simulink model "Citation"  (Simulink 10.1)
settings: Solver=ode5  StartTime=0.0  StopTime=inf  FixedStep=0.01  RelTol=1e-3  EnableMultiTasking=on
values from neighbouring files (symbols this model uses):
  S = 12.9900    (= 12.99)    [FTFC.m]
  Vw915 = 0    [initcit.m]
  winddir = 45*(pi/180)    (= 0.785398163397)    [initcit.m]
  x0 = []    [cessnac550_3d_sfnc.m]    (also in sfunxyz.m)
undefined symbols (not defined in the file or in its folder): chord, cv1, cv2, cv3, cv4, deltagmax1, deltagmax2, deltagmax3, deltagmax4, Deng, ealphag, ealphas, g0, hDME, hGS, kt1, kt2, kt3, lh, massinit, matbuaf, matdaf, matdam, matdbbf, matdeaf, matdgaf, matdqaf, matduaf, matdwaw, matedhr, mateif, matelhr, matemhr, matemv1, matemv2, matemve, matetam, mateuaf, matfaaf, matfaxl, matff, matibaf, matibmh, matipaf, matipmh, matiraf, matiuaf, matiwaf, matlaf, matlam, matleaf, matleam, matlgaf, matlqaf, matluaf, matmaaf, matmaam, matmaf, matmam, matmbbf ... (+74)
undefined symbols (not defined in the file): matibb
libraries: simulink x12, vrlib x1
(part 5 of 5)

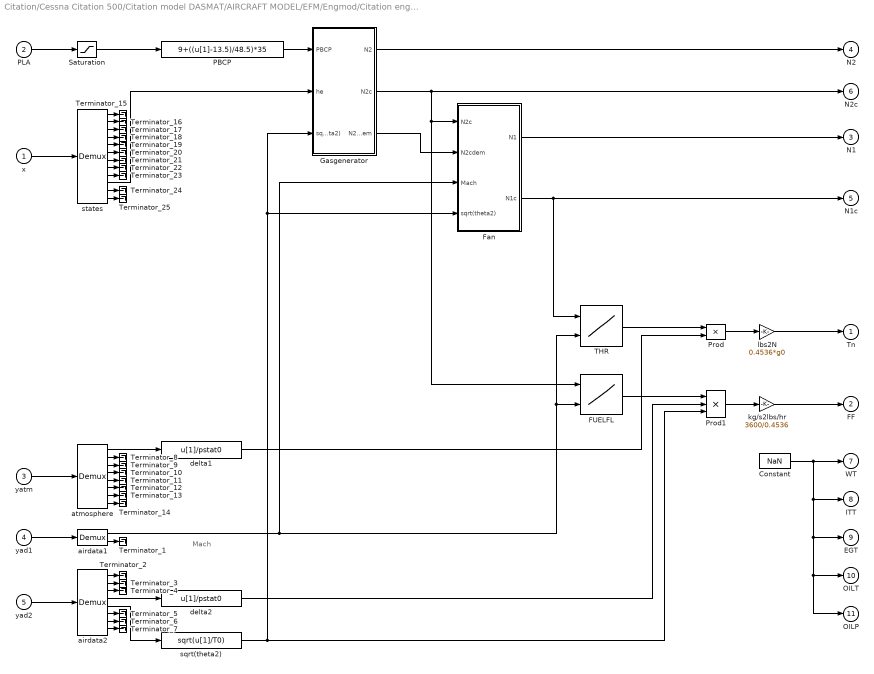
== system Citation/Cessna Citation 500/Citation model DASMAT/AIRCRAFT MODEL/EFM/Engmod/Citation eng_mod/Subsystem1/JT15 Dynamic/Subsystem/engine ==
  note: Mach
  x : Inport
  PLA : Inport  Port=2
  yatm : Inport  Port=3
  yad1 : Inport  Port=4
  yad2 : Inport  Port=5
  Constant : Constant  Value=NaN
  FUELFL : Lookup2D  RowIndex=matff(2:14,1)  ColumnIndex=matff(1,2:14)  Table=matff(2:14,2:14)  SaturateOnIntegerOverflow=on  InputSameDT=on
  Fan : Subsystem
  Gasgenerator : Subsystem
  PBCP : Fcn  Expr=9+((u[1]-13.5)/48.5)*35
  Prod : Product  InputSameDT=on  SaturateOnIntegerOverflow=on  OutDataTypeStr=Inherit: Same as first input
  Prod1 : Product  Inputs=3  InputSameDT=on  SaturateOnIntegerOverflow=on  OutDataTypeStr=Inherit: Same as first input
  Saturation : Saturate  UpperLimit=62  LowerLimit=13.5
  THR : Lookup2D  RowIndex=matthr(2:12,1)  ColumnIndex=matthr(1,2:12)  Table=matthr(2:12,2:12)  SaturateOnIntegerOverflow=on  InputSameDT=on
  Terminator_{1..25} (25 alike) : Terminator
  airdata1 : Demux  Outputs=2
      settings: DisplayOption=none
  airdata2 : Demux  Outputs=8
      settings: DisplayOption=none
  atmosphere : Demux  Outputs=8
      settings: DisplayOption=none
  delta1 : Fcn  Expr=u[1]/pstat0
  delta2 : Fcn  Expr=u[1]/pstat0
  kg/s2lbs/hr : Gain  Gain=3600/0.4536  SaturateOnIntegerOverflow=on  OutDataTypeStr=Inherit: Same as input  ParamDataTypeStr=Inherit: Same as input
  lbs2N : Gain  Gain=0.4536*g0  SaturateOnIntegerOverflow=on  OutDataTypeStr=Inherit: Same as input  ParamDataTypeStr=Inherit: Same as input
  sqrt(theta2) : Fcn  Expr=sqrt(u[1]/T0)
  states : Demux  Outputs=12
      settings: DisplayOption=none
  Tn : Outport
  FF : Outport  Port=2
  N1 : Outport  Port=3
  N2 : Outport  Port=4
  N1c : Outport  Port=5
  N2c : Outport  Port=6
  WT : Outport  Port=7
  ITT : Outport  Port=8
  EGT : Outport  Port=9
  OILT : Outport  Port=10
  OILP : Outport  Port=11
  wires:
  states/12 -> Terminator_25/1
  states/11 -> Terminator_24/1
  states/9 -> Terminator_23/1
  states/8 -> Terminator_22/1
  states/7 -> Terminator_21/1
  states/6 -> Terminator_20/1
  states/5 -> Terminator_19/1
  states/4 -> Terminator_18/1
  states/3 -> Terminator_17/1
  states/2 -> Terminator_16/1
  states/1 -> Terminator_15/1
  atmosphere/8 -> Terminator_14/1
  atmosphere/7 -> Terminator_13/1
  atmosphere/6 -> Terminator_12/1
  atmosphere/5 -> Terminator_11/1
  atmosphere/4 -> Terminator_10/1
  atmosphere/3 -> Terminator_9/1
  atmosphere/2 -> Terminator_8/1
  airdata2/8 -> Terminator_7/1
  airdata2/7 -> Terminator_6/1
  airdata2/6 -> Terminator_5/1
  airdata2/3 -> Terminator_4/1
  airdata2/2 -> Terminator_3/1
  airdata2/1 -> Terminator_2/1
  airdata1/2 -> Terminator_1/1
  Fan/2(N1c) -> THR/1, N1c/1
  Gasgenerator/2(N2c) -> Fan/1(N2c), FUELFL/1, N2c/1
  Gasgenerator/3(N2cdem) -> Fan/2(N2cdem)
  airdata1/1 -> Fan/3(Mach), FUELFL/2, THR/2
  Fan/1(N1) -> N1/1
  sqrt(theta2)/1 -> Fan/4(sqrt(theta2)), Gasgenerator/3(sqrt(theta2)), Prod1/3
  yad2/1 -> airdata2/1
  yad1/1 -> airdata1/1
  yatm/1 -> atmosphere/1
  airdata2/4 -> delta2/1
  airdata2/5 -> sqrt(theta2)/1
  Constant/1 -> ITT/1, EGT/1, OILT/1, OILP/1, WT/1
  Gasgenerator/1(N2) -> N2/1
  delta1/1 -> Prod/2
  Prod/1 -> lbs2N/1
  THR/1 -> Prod/1
  lbs2N/1 -> Tn/1
  states/10 -> Gasgenerator/2(he)
  delta2/1 -> Prod1/2
  atmosphere/1 -> delta1/1
  Prod1/1 -> kg/s2lbs/hr/1
  kg/s2lbs/hr/1 -> FF/1
  Saturation/1 -> PBCP/1
  PLA/1 -> Saturation/1
  x/1 -> states/1
  PBCP/1 -> Gasgenerator/1(PBCP)
  FUELFL/1 -> Prod1/1

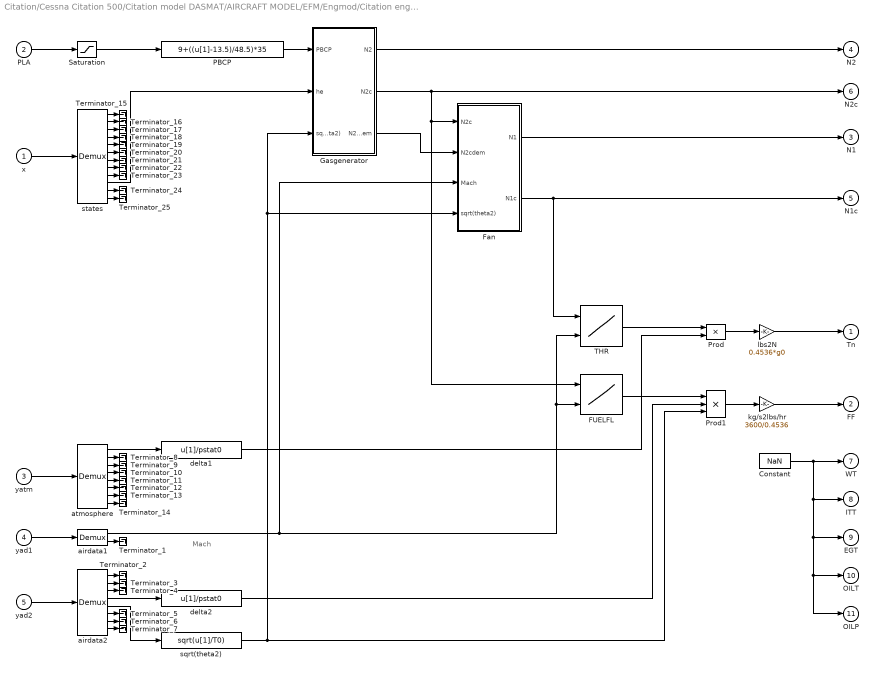
== system Citation/Cessna Citation 500/Citation model DASMAT/AIRCRAFT MODEL/EFM/Engmod/Citation eng_mod/Subsystem1/JT15 Dynamic1/Subsystem/engine ==
  note: Mach
  x : Inport
  PLA : Inport  Port=2
  yatm : Inport  Port=3
  yad1 : Inport  Port=4
  yad2 : Inport  Port=5
  Constant : Constant  Value=NaN
  FUELFL : Lookup2D  RowIndex=matff(2:14,1)  ColumnIndex=matff(1,2:14)  Table=matff(2:14,2:14)  SaturateOnIntegerOverflow=on  InputSameDT=on
  Fan : Subsystem
  Gasgenerator : Subsystem
  PBCP : Fcn  Expr=9+((u[1]-13.5)/48.5)*35
  Prod : Product  InputSameDT=on  SaturateOnIntegerOverflow=on  OutDataTypeStr=Inherit: Same as first input
  Prod1 : Product  Inputs=3  InputSameDT=on  SaturateOnIntegerOverflow=on  OutDataTypeStr=Inherit: Same as first input
  Saturation : Saturate  UpperLimit=62  LowerLimit=13.5
  THR : Lookup2D  RowIndex=matthr(2:12,1)  ColumnIndex=matthr(1,2:12)  Table=matthr(2:12,2:12)  SaturateOnIntegerOverflow=on  InputSameDT=on
  Terminator_{1..25} (25 alike) : Terminator
  airdata1 : Demux  Outputs=2
      settings: DisplayOption=none
  airdata2 : Demux  Outputs=8
      settings: DisplayOption=none
  atmosphere : Demux  Outputs=8
      settings: DisplayOption=none
  delta1 : Fcn  Expr=u[1]/pstat0
  delta2 : Fcn  Expr=u[1]/pstat0
  kg/s2lbs/hr : Gain  Gain=3600/0.4536  SaturateOnIntegerOverflow=on  OutDataTypeStr=Inherit: Same as input  ParamDataTypeStr=Inherit: Same as input
  lbs2N : Gain  Gain=0.4536*g0  SaturateOnIntegerOverflow=on  OutDataTypeStr=Inherit: Same as input  ParamDataTypeStr=Inherit: Same as input
  sqrt(theta2) : Fcn  Expr=sqrt(u[1]/T0)
  states : Demux  Outputs=12
      settings: DisplayOption=none
  Tn : Outport
  FF : Outport  Port=2
  N1 : Outport  Port=3
  N2 : Outport  Port=4
  N1c : Outport  Port=5
  N2c : Outport  Port=6
  WT : Outport  Port=7
  ITT : Outport  Port=8
  EGT : Outport  Port=9
  OILT : Outport  Port=10
  OILP : Outport  Port=11
  wires:
  states/12 -> Terminator_25/1
  states/11 -> Terminator_24/1
  states/9 -> Terminator_23/1
  states/8 -> Terminator_22/1
  states/7 -> Terminator_21/1
  states/6 -> Terminator_20/1
  states/5 -> Terminator_19/1
  states/4 -> Terminator_18/1
  states/3 -> Terminator_17/1
  states/2 -> Terminator_16/1
  states/1 -> Terminator_15/1
  atmosphere/8 -> Terminator_14/1
  atmosphere/7 -> Terminator_13/1
  atmosphere/6 -> Terminator_12/1
  atmosphere/5 -> Terminator_11/1
  atmosphere/4 -> Terminator_10/1
  atmosphere/3 -> Terminator_9/1
  atmosphere/2 -> Terminator_8/1
  airdata2/8 -> Terminator_7/1
  airdata2/7 -> Terminator_6/1
  airdata2/6 -> Terminator_5/1
  airdata2/3 -> Terminator_4/1
  airdata2/2 -> Terminator_3/1
  airdata2/1 -> Terminator_2/1
  airdata1/2 -> Terminator_1/1
  Fan/2(N1c) -> THR/1, N1c/1
  Gasgenerator/2(N2c) -> Fan/1(N2c), FUELFL/1, N2c/1
  Gasgenerator/3(N2cdem) -> Fan/2(N2cdem)
  airdata1/1 -> Fan/3(Mach), FUELFL/2, THR/2
  Fan/1(N1) -> N1/1
  sqrt(theta2)/1 -> Fan/4(sqrt(theta2)), Gasgenerator/3(sqrt(theta2)), Prod1/3
  yad2/1 -> airdata2/1
  yad1/1 -> airdata1/1
  yatm/1 -> atmosphere/1
  airdata2/4 -> delta2/1
  airdata2/5 -> sqrt(theta2)/1
  Constant/1 -> ITT/1, EGT/1, OILT/1, OILP/1, WT/1
  Gasgenerator/1(N2) -> N2/1
  delta1/1 -> Prod/2
  Prod/1 -> lbs2N/1
  THR/1 -> Prod/1
  lbs2N/1 -> Tn/1
  states/10 -> Gasgenerator/2(he)
  delta2/1 -> Prod1/2
  atmosphere/1 -> delta1/1
  Prod1/1 -> kg/s2lbs/hr/1
  kg/s2lbs/hr/1 -> FF/1
  Saturation/1 -> PBCP/1
  PLA/1 -> Saturation/1
  x/1 -> states/1
  PBCP/1 -> Gasgenerator/1(PBCP)
  FUELFL/1 -> Prod1/1

== system Citation/Cessna Citation 500/Citation model DASMAT/AIRCRAFT MODEL/EFM/Engmod/Citation eng_mod/Subsystem1/JT15 Dynamic/Subsystem/engine/Fan ==
  note: N1c feedback
  note: N1cdot
  N2c : Inport
  N2cdem : Inport  Port=2
  Mach : Inport  Port=3
  sqrt(theta2) : Inport  Port=4
  Droop : Gain  Gain=2  SaturateOnIntegerOverflow=on  OutDataTypeStr=Inherit: Same as input  ParamDataTypeStr=Inherit: Same as input
  Max accel : Subsystem  mask(Min Value){}
      mask help:
      | Output is minimum value of inputs.
      | y=min(u1,u2)
      mask Help: The Min block produces as output the minimum value of two scalars or vectors. If the inputs are vectors, the output will be a vector containing the minimum elements of the vectors.
      mask Display: disp('Min')
  Max decel : Subsystem  mask(Max Value){}
      mask help:
      | Output is maximum value of inputs.
      | y=max(u1,u2)
      mask Help: The Max block produces as output the maximum value of two scalars or vectors. If the inputs are vectors, the output will be a vector containing the maximum elements of the vectors.
      mask Display: disp('Max')
  N1 state : Integrator  InitialCondition=xt0(2)
  N1D : Lookup2D  RowIndex=matn1d(2:14,1)  ColumnIndex=matn1d(1,2:14)  Table=matn1d(2:14,2:14)  SaturateOnIntegerOverflow=on  InputSameDT=on
  Prod : Product  InputSameDT=on  SaturateOnIntegerOverflow=on  OutDataTypeStr=Inherit: Same as first input
  Sum : Sum  Inputs=+-  InputSameDT=on  SaturateOnIntegerOverflow=on  OutDataTypeStr=Inherit: Same as first input
  fN1cmax : Lookup  InputValues="[0 25 40 70 94  120]"  Table="[0   0   1   12 14  18]"  SaturateOnIntegerOverflow=on
  fN1cmin : Lookup  InputValues="[25     50   60   94 100]"  Table="[-0.05  -0.05    -1    -30 -28]"  SaturateOnIntegerOverflow=on
  N1 : Outport
  N1c : Outport  Port=2
  wires:
  sqrt(theta2)/1 -> Prod/2
  N1 state/1 -> Prod/1, Sum/2, N1c/1
  N2c/1 -> fN1cmin/1, fN1cmax/1
  Max decel/1(out_1) -> N1 state/1
  N1D/1 -> Sum/1
  Max accel/1(out_1) -> Max decel/1(in_1)
  fN1cmax/1 -> Max accel/2(in_2)
  fN1cmin/1 -> Max decel/2(in_2)
  Sum/1 -> Droop/1
  Droop/1 -> Max accel/1(in_1)
  Mach/1 -> N1D/2
  Prod/1 -> N1/1
  N2cdem/1 -> N1D/1

== system Citation/Cessna Citation 500/Citation model DASMAT/AIRCRAFT MODEL/EFM/Engmod/Citation eng_mod/Subsystem1/JT15 Dynamic/Subsystem/engine/Gasgenerator ==
  note: N2 feedback
  note: N2dot
  PBCP : Inport
  he : Inport  Port=2
  sqrt(theta2) : Inport  Port=3
  Droop : Lookup  InputValues=[0 100]  Table="[0.1  2]"  SaturateOnIntegerOverflow=on
  Fcn : Fcn  Expr=u[1]/u[2]
  Fcn1 : Fcn  Expr=u[1]/u[2]
  Governor : Product  InputSameDT=on  SaturateOnIntegerOverflow=on  OutDataTypeStr=Inherit: Same as first input
  Max accel : Subsystem  mask(Max Value){}
      mask help:
      | Output is maximum value of inputs.
      | y=max(u1,u2)
      mask Help: The Max block produces as output the maximum value of two scalars or vectors. If the inputs are vectors, the output will be a vector containing the maximum elements of the vectors.
      mask Display: disp('Max')
  Min accel : Subsystem  mask(Min Value){}
      mask help:
      | Output is minimum value of inputs.
      | y=min(u1,u2)
      mask Help: The Min block produces as output the minimum value of two scalars or vectors. If the inputs are vectors, the output will be a vector containing the minimum elements of the vectors.
      mask Display: disp('Min')
  Mux : Mux  Inputs=2
  Mux1 : Mux  Inputs=2
  N2 state : Integrator  InitialCondition=xt0(1)
  N2D : Lookup2D  RowIndex=matn2d(2:10,1)  ColumnIndex=matn2d(1,2:10)  Table=matn2d(2:10,2:10)  SaturateOnIntegerOverflow=on  InputSameDT=on
  Sum : Sum  Inputs=+-  InputSameDT=on  SaturateOnIntegerOverflow=on  OutDataTypeStr=Inherit: Same as first input
  fN2max : Lookup  InputValues=[25 40 70 94]  Table=[0 3 8 10]  SaturateOnIntegerOverflow=on
  fN2min : Lookup  InputValues="[25     50   60   94 100]"  Table="[-0.05  -0.05    -2    -20 -28]"  SaturateOnIntegerOverflow=on
  ft2FL : Gain  Gain=.01  SaturateOnIntegerOverflow=on  OutDataTypeStr=Inherit: Same as input  ParamDataTypeStr=Inherit: Same as input
  m2ft : Gain  Gain=(1/0.3048)  SaturateOnIntegerOverflow=on  OutDataTypeStr=Inherit: Same as input  ParamDataTypeStr=Inherit: Same as input
  N2 : Outport
  N2c : Outport  Port=2
  N2cdem : Outport  Port=3
  wires:
  sqrt(theta2)/1 -> Mux1/2, Mux/2
  N2D/1 -> Mux/1, Droop/1, Sum/1
  Fcn1/1 -> N2c/1
  Fcn/1 -> N2cdem/1
  Mux1/1 -> Fcn1/1
  Mux/1 -> Fcn/1
  Min accel/1(out_1) -> Max accel/1(in_1)
  ft2FL/1 -> N2D/2
  m2ft/1 -> ft2FL/1
  he/1 -> m2ft/1
  N2 state/1 -> Mux1/1, fN2min/1, fN2max/1, Sum/2, N2/1
  fN2max/1 -> Min accel/2(in_2)
  fN2min/1 -> Max accel/2(in_2)
  PBCP/1 -> N2D/1
  Droop/1 -> Governor/1
  Sum/1 -> Governor/2
  Governor/1 -> Min accel/1(in_1)
  Max accel/1(out_1) -> N2 state/1

== system Citation/Cessna Citation 500/Citation model DASMAT/AIRCRAFT MODEL/EFM/Engmod/Citation eng_mod/Subsystem1/JT15 Dynamic1/Subsystem/engine/Fan ==
  note: N1c feedback
  note: N1cdot
  N2c : Inport
  N2cdem : Inport  Port=2
  Mach : Inport  Port=3
  sqrt(theta2) : Inport  Port=4
  Droop : Gain  Gain=2  SaturateOnIntegerOverflow=on  OutDataTypeStr=Inherit: Same as input  ParamDataTypeStr=Inherit: Same as input
  Max accel : Subsystem  mask(Min Value){}
      mask help:
      | Output is minimum value of inputs.
      | y=min(u1,u2)
      mask Help: The Min block produces as output the minimum value of two scalars or vectors. If the inputs are vectors, the output will be a vector containing the minimum elements of the vectors.
      mask Display: disp('Min')
  Max decel : Subsystem  mask(Max Value){}
      mask help:
      | Output is maximum value of inputs.
      | y=max(u1,u2)
      mask Help: The Max block produces as output the maximum value of two scalars or vectors. If the inputs are vectors, the output will be a vector containing the maximum elements of the vectors.
      mask Display: disp('Max')
  N1 state : Integrator  InitialCondition=xt0(2)
  N1D : Lookup2D  RowIndex=matn1d(2:14,1)  ColumnIndex=matn1d(1,2:14)  Table=matn1d(2:14,2:14)  SaturateOnIntegerOverflow=on  InputSameDT=on
  Prod : Product  InputSameDT=on  SaturateOnIntegerOverflow=on  OutDataTypeStr=Inherit: Same as first input
  Sum : Sum  Inputs=+-  InputSameDT=on  SaturateOnIntegerOverflow=on  OutDataTypeStr=Inherit: Same as first input
  fN1cmax : Lookup  InputValues="[0 25 40 70 94  120]"  Table="[0   0   1   12 14  18]"  SaturateOnIntegerOverflow=on
  fN1cmin : Lookup  InputValues="[25     50   60   94 100]"  Table="[-0.05  -0.05    -1    -30 -28]"  SaturateOnIntegerOverflow=on
  N1 : Outport
  N1c : Outport  Port=2
  wires:
  sqrt(theta2)/1 -> Prod/2
  N1 state/1 -> Prod/1, Sum/2, N1c/1
  N2c/1 -> fN1cmin/1, fN1cmax/1
  Max decel/1(out_1) -> N1 state/1
  N1D/1 -> Sum/1
  Max accel/1(out_1) -> Max decel/1(in_1)
  fN1cmax/1 -> Max accel/2(in_2)
  fN1cmin/1 -> Max decel/2(in_2)
  Sum/1 -> Droop/1
  Droop/1 -> Max accel/1(in_1)
  Mach/1 -> N1D/2
  Prod/1 -> N1/1
  N2cdem/1 -> N1D/1

== system Citation/Cessna Citation 500/Citation model DASMAT/AIRCRAFT MODEL/EFM/Engmod/Citation eng_mod/Subsystem1/JT15 Dynamic1/Subsystem/engine/Gasgenerator ==
  note: N2 feedback
  note: N2dot
  PBCP : Inport
  he : Inport  Port=2
  sqrt(theta2) : Inport  Port=3
  Droop : Lookup  InputValues=[0 100]  Table="[0.1  2]"  SaturateOnIntegerOverflow=on
  Fcn : Fcn  Expr=u[1]/u[2]
  Fcn1 : Fcn  Expr=u[1]/u[2]
  Governor : Product  InputSameDT=on  SaturateOnIntegerOverflow=on  OutDataTypeStr=Inherit: Same as first input
  Max accel : Subsystem  mask(Max Value){}
      mask help:
      | Output is maximum value of inputs.
      | y=max(u1,u2)
      mask Help: The Max block produces as output the maximum value of two scalars or vectors. If the inputs are vectors, the output will be a vector containing the maximum elements of the vectors.
      mask Display: disp('Max')
  Min accel : Subsystem  mask(Min Value){}
      mask help:
      | Output is minimum value of inputs.
      | y=min(u1,u2)
      mask Help: The Min block produces as output the minimum value of two scalars or vectors. If the inputs are vectors, the output will be a vector containing the minimum elements of the vectors.
      mask Display: disp('Min')
  Mux : Mux  Inputs=2
  Mux1 : Mux  Inputs=2
  N2 state : Integrator  InitialCondition=xt0(1)
  N2D : Lookup2D  RowIndex=matn2d(2:10,1)  ColumnIndex=matn2d(1,2:10)  Table=matn2d(2:10,2:10)  SaturateOnIntegerOverflow=on  InputSameDT=on
  Sum : Sum  Inputs=+-  InputSameDT=on  SaturateOnIntegerOverflow=on  OutDataTypeStr=Inherit: Same as first input
  fN2max : Lookup  InputValues=[25 40 70 94]  Table=[0 3 8 10]  SaturateOnIntegerOverflow=on
  fN2min : Lookup  InputValues="[25     50   60   94 100]"  Table="[-0.05  -0.05    -2    -20 -28]"  SaturateOnIntegerOverflow=on
  ft2FL : Gain  Gain=.01  SaturateOnIntegerOverflow=on  OutDataTypeStr=Inherit: Same as input  ParamDataTypeStr=Inherit: Same as input
  m2ft : Gain  Gain=(1/0.3048)  SaturateOnIntegerOverflow=on  OutDataTypeStr=Inherit: Same as input  ParamDataTypeStr=Inherit: Same as input
  N2 : Outport
  N2c : Outport  Port=2
  N2cdem : Outport  Port=3
  wires:
  sqrt(theta2)/1 -> Mux1/2, Mux/2
  N2D/1 -> Mux/1, Droop/1, Sum/1
  Fcn1/1 -> N2c/1
  Fcn/1 -> N2cdem/1
  Mux1/1 -> Fcn1/1
  Mux/1 -> Fcn/1
  Min accel/1(out_1) -> Max accel/1(in_1)
  ft2FL/1 -> N2D/2
  m2ft/1 -> ft2FL/1
  he/1 -> m2ft/1
  N2 state/1 -> Mux1/1, fN2min/1, fN2max/1, Sum/2, N2/1
  fN2max/1 -> Min accel/2(in_2)
  fN2min/1 -> Max accel/2(in_2)
  PBCP/1 -> N2D/1
  Droop/1 -> Governor/1
  Sum/1 -> Governor/2
  Governor/1 -> Min accel/1(in_1)
  Max accel/1(out_1) -> N2 state/1

== system Citation/Cessna Citation 500/Citation model DASMAT/AIRCRAFT MODEL/EFM/Engmod/Citation eng_mod/Subsystem1/JT15 Dynamic/Subsystem/engine/Fan/Max accel ==
  in_1 : Inport
  in_2 : Inport  Port=2
  Sum : Sum  Inputs=-+  InputSameDT=on  SaturateOnIntegerOverflow=on  OutDataTypeStr=Inherit: Same as first input
  Switch : Switch  SaturateOnIntegerOverflow=on  InputSameDT=on
  out_1 : Outport
  wires:
  in_1/1 -> Sum/1, Switch/1
  in_2/1 -> Sum/2, Switch/3
  Sum/1 -> Switch/2
  Switch/1 -> out_1/1

== system Citation/Cessna Citation 500/Citation model DASMAT/AIRCRAFT MODEL/EFM/Engmod/Citation eng_mod/Subsystem1/JT15 Dynamic/Subsystem/engine/Fan/Max decel ==
  in_1 : Inport
  in_2 : Inport  Port=2
  Sum : Sum  Inputs=+-  InputSameDT=on  SaturateOnIntegerOverflow=on  OutDataTypeStr=Inherit: Same as first input
  Switch : Switch  SaturateOnIntegerOverflow=on  InputSameDT=on
  out_1 : Outport
  wires:
  Switch/1 -> out_1/1
  Sum/1 -> Switch/2
  in_2/1 -> Sum/2, Switch/3
  in_1/1 -> Sum/1, Switch/1

== system Citation/Cessna Citation 500/Citation model DASMAT/AIRCRAFT MODEL/EFM/Engmod/Citation eng_mod/Subsystem1/JT15 Dynamic/Subsystem/engine/Gasgenerator/Max accel ==
  in_1 : Inport
  in_2 : Inport  Port=2
  Sum : Sum  Inputs=+-  InputSameDT=on  SaturateOnIntegerOverflow=on  OutDataTypeStr=Inherit: Same as first input
  Switch : Switch  SaturateOnIntegerOverflow=on  InputSameDT=on
  out_1 : Outport
  wires:
  Switch/1 -> out_1/1
  Sum/1 -> Switch/2
  in_2/1 -> Sum/2, Switch/3
  in_1/1 -> Sum/1, Switch/1

== system Citation/Cessna Citation 500/Citation model DASMAT/AIRCRAFT MODEL/EFM/Engmod/Citation eng_mod/Subsystem1/JT15 Dynamic/Subsystem/engine/Gasgenerator/Min accel ==
  in_1 : Inport
  in_2 : Inport  Port=2
  Sum : Sum  Inputs=-+  InputSameDT=on  SaturateOnIntegerOverflow=on  OutDataTypeStr=Inherit: Same as first input
  Switch : Switch  SaturateOnIntegerOverflow=on  InputSameDT=on
  out_1 : Outport
  wires:
  in_1/1 -> Sum/1, Switch/1
  in_2/1 -> Sum/2, Switch/3
  Sum/1 -> Switch/2
  Switch/1 -> out_1/1

== system Citation/Cessna Citation 500/Citation model DASMAT/AIRCRAFT MODEL/EFM/Engmod/Citation eng_mod/Subsystem1/JT15 Dynamic1/Subsystem/engine/Fan/Max accel ==
  in_1 : Inport
  in_2 : Inport  Port=2
  Sum : Sum  Inputs=-+  InputSameDT=on  SaturateOnIntegerOverflow=on  OutDataTypeStr=Inherit: Same as first input
  Switch : Switch  SaturateOnIntegerOverflow=on  InputSameDT=on
  out_1 : Outport
  wires:
  in_1/1 -> Sum/1, Switch/1
  in_2/1 -> Sum/2, Switch/3
  Sum/1 -> Switch/2
  Switch/1 -> out_1/1

== system Citation/Cessna Citation 500/Citation model DASMAT/AIRCRAFT MODEL/EFM/Engmod/Citation eng_mod/Subsystem1/JT15 Dynamic1/Subsystem/engine/Fan/Max decel ==
  in_1 : Inport
  in_2 : Inport  Port=2
  Sum : Sum  Inputs=+-  InputSameDT=on  SaturateOnIntegerOverflow=on  OutDataTypeStr=Inherit: Same as first input
  Switch : Switch  SaturateOnIntegerOverflow=on  InputSameDT=on
  out_1 : Outport
  wires:
  Switch/1 -> out_1/1
  Sum/1 -> Switch/2
  in_2/1 -> Sum/2, Switch/3
  in_1/1 -> Sum/1, Switch/1

== system Citation/Cessna Citation 500/Citation model DASMAT/AIRCRAFT MODEL/EFM/Engmod/Citation eng_mod/Subsystem1/JT15 Dynamic1/Subsystem/engine/Gasgenerator/Max accel ==
  in_1 : Inport
  in_2 : Inport  Port=2
  Sum : Sum  Inputs=+-  InputSameDT=on  SaturateOnIntegerOverflow=on  OutDataTypeStr=Inherit: Same as first input
  Switch : Switch  SaturateOnIntegerOverflow=on  InputSameDT=on
  out_1 : Outport
  wires:
  Switch/1 -> out_1/1
  Sum/1 -> Switch/2
  in_2/1 -> Sum/2, Switch/3
  in_1/1 -> Sum/1, Switch/1

== system Citation/Cessna Citation 500/Citation model DASMAT/AIRCRAFT MODEL/EFM/Engmod/Citation eng_mod/Subsystem1/JT15 Dynamic1/Subsystem/engine/Gasgenerator/Min accel ==
  in_1 : Inport
  in_2 : Inport  Port=2
  Sum : Sum  Inputs=-+  InputSameDT=on  SaturateOnIntegerOverflow=on  OutDataTypeStr=Inherit: Same as first input
  Switch : Switch  SaturateOnIntegerOverflow=on  InputSameDT=on
  out_1 : Outport
  wires:
  in_1/1 -> Sum/1, Switch/1
  in_2/1 -> Sum/2, Switch/3
  Sum/1 -> Switch/2
  Switch/1 -> out_1/1

== matlab function Aerodynamic Model Identification/Autocorrelation ==
  data: correlation output double; Inputs input double; C_list1 input double; C_list1 output double
function [correlation, C_list1] = autocorr(Inputs, C_list1)
%% Define Window Size
window = 100;
k_gap  = [0,10,20,30,40,50,60,70,80,90];

%% Define Aerodynamic Matrix
C_list_new = C_list1(:,2:end);
C_list_new = horzcat(C_list_new, Inputs);

%% Calculate Autocorrelation
corr1 = (1/window) * sum(C_list_new(:,1:end-k_gap(1)).*C_list_new(:,k_gap(1)+1:end),2);
corr2 = (1/window) * sum(C_list_new(:,1:end-k_gap(2)).*C_list_new(:,k_gap(2)+1:end),2);
corr3 = (1/window) * sum(C_list_new(:,1:end-k_gap(3)).*C_list_new(:,k_gap(3)+1:end),2);
corr4 = (1/window) * sum(C_list_new(:,1:end-k_gap(4)).*C_list_new(:,k_gap(4)+1:end),2);
corr5 = (1/window) * sum(C_list_new(:,1:end-k_gap(5)).*C_list_new(:,k_gap(5)+1:end),2);
corr6 = (1/window) * sum(C_list_new(:,1:end-k_gap(6)).*C_list_new(:,k_gap(6)+1:end),2);
corr7 = (1/window) * sum(C_list_new(:,1:end-k_gap(7)).*C_list_new(:,k_gap(7)+1:end),2);
corr8 = (1/window) * sum(C_list_new(:,1:end-k_gap(8)).*C_list_new(:,k_gap(8)+1:end),2);
corr9 = (1/window) * sum(C_list_new(:,1:end-k_gap(9)).*C_list_new(:,k_gap(9)+1:end),2);
corr10 = (1/window) * sum(C_list_new(:,1:end-k_gap(10)).*C_list_new(:,k_gap(10)+1:end),2);

%% Calculate Confidence Interval
conf = (1.95*corr1)/sqrt(window);


%% Update Matrix
C_list1 = C_list_new;
correlation = [corr1;corr2;corr3;corr4;corr5;corr6;corr7;corr8;corr9;corr10;conf];

== matlab function Aerodynamic Model Identification/Recursive Least Square ==
  data: Inputs input double; y output double; P1 input double; P2 input double; P3 input double; P4 input double; P5 input double; P6 input double; p_est1 input double; y_est output double; P1 output double; P2 output double; P3 output double; P4 output double; P5 output double; P6 output double; p_est1 output double; p_est2 input double; p_est3 input double; p_est4 input double; p_est5 input double; p_est6 input double; p_est2 output double; p_est3 output double; p_est4 output double; p_est5 output double; p_est6 output double; rho output double; C_innovation input double; C_innovation output double; trigger input double; trigger output double; var_old output double; var_old input double
function [y,y_est,P1,P2,P3,P4,P5,P6,p_est1,p_est2,p_est3,p_est4,p_est5,p_est6,rho, C_innovation, trigger, var_old] =...
    RLS(Inputs,P1,P2,P3,P4,P5,P6,p_est1,p_est2,p_est3,p_est4, ...
    p_est5,p_est6, C_innovation, trigger,var_old)
%% Initialize aircraft and atmospheric parameters
Ixx = 11187.8;   b = 13.3250;    R       = 287.05;    rho0    = 1.225;
Iyy = 22854.8;   S = 24.9900;    ltrop   = -0.0065;   htropo  = 11000;
Izz = 31974.8;   c = 1.9910;     h0      = 0;         hstrato = 20000;
Ixz = 1930.1;    m = 4500;       T0      = 288.15;    g       = 9.80665;

%% Define reset covariance matrix
Pr_1 = eye(5) * 10000;
Pr_2 = eye(4) * 10000;
Pr_3 = eye(4) * 10000;
Pr_4 = eye(6) * 10000;
Pr_5 = eye(6) * 10000;
Pr_6 = eye(6) * 10000;

% Reset covariance matrix Y, l and n channel in case of failure
if trigger == 0
        P4 = Pr_4;
        P5 = Pr_5;
        P6 = Pr_6;
end

%% Forgetting factor
lambda = 1;

%% Initialize state parameters
p       = Inputs(1);    he      = Inputs(7);    anxb    = Inputs(13)*g;
q       = Inputs(2);    xe      = Inputs(8);    anyb    = Inputs(14)*g;
r       = Inputs(3);    ye      = Inputs(9);    anzb    = Inputs(15)*g;
vtas    = Inputs(4);    p_dot   = Inputs(10);   de      = Inputs(16);
alpha   = Inputs(5);    q_dot   = Inputs(11);   da      = Inputs(17);
beta    = Inputs(6);    r_dot   = Inputs(12);   dr      = Inputs(18);

%% Atmospheric calculations
if he > htropo
    rho_tropo = rho0 * (1+ltrop*(htropo/T0))^(-(g/(R*ltrop))-1);    
    T_tropo = T0 + (htropo - h0)*ltrop;                             
    rho = rho_tropo + rho_tropo * exp(-(g/(R*T_tropo))*(he-htropo));
else
    rho = rho0 * (1+ltrop*(he/T0))^(-(g/(R*ltrop))-1);              
end

%% Aerodynamic forces and moment calculations
Cx = (m*anxb) / (0.5*rho*vtas^2*S); L = p_dot*Ixx + q*r*(Izz-Iyy) - (p*q + r_dot)*Ixz; 
Cy = (m*anyb) / (0.5*rho*vtas^2*S); M = q_dot*Iyy + r*p*(Ixx-Izz) + (p*p - r*r)*Ixz;    
Cz = (m*anzb) / (0.5*rho*vtas^2*S); N = r_dot*Izz + p*q*(Iyy-Ixx) + (q*r - p_dot)*Ixz;

Cl = L / (0.5*rho*vtas^2*S*b); 
Cm = M / (0.5*rho*vtas^2*S*c); 
Cn = N / (0.5*rho*vtas^2*S*b); 

y1 = Cx;    y4 = Cy;
y2 = Cz;    y5 = Cl;
y3 = Cm;    y6 = Cn;

%% Initialize regression matrix
H_y1 = [1; alpha; alpha^2; (q*c/vtas); de]; 
H_y2 = [1; alpha; (q*c/vtas); de];          
H_y3 = [1; alpha; (q*c/vtas); de];          

H_y4 = [1; beta; (p*b/2*vtas); (r*b/2*vtas); da; de]; 
H_y5 = [1; beta; (p*b/2*vtas); (r*b/2*vtas); da; de];
H_y6 = [1; beta; (p*b/2*vtas); (r*b/2*vtas); da; de];

%% Intialize parameters estimate
p_1 = p_est1;
p_2 = p_est2;
p_3 = p_est3;
p_4 = p_est4;
p_5 = p_est5;
p_6 = p_est6;

%% Calculate least square estimate
L_k1 = P1*H_y1 * inv(H_y1'*P1*H_y1 + lambda);
L_k2 = P2*H_y2 * inv(H_y2'*P2*H_y2 + lambda);
L_k3 = P3*H_y3 * inv(H_y3'*P3*H_y3 + lambda);
L_k4 = P4*H_y4 * inv(H_y4'*P4*H_y4 + lambda);
L_k5 = P5*H_y5 * inv(H_y5'*P5*H_y5 + lambda);
L_k6 = P6*H_y6 * inv(H_y6'*P6*H_y6 + lambda);

%% Update parameter
p_k1 = p_1 + L_k1*(y1 - H_y1'*p_1);
p_k2 = p_2 + L_k2*(y2 - H_y2'*p_2);
p_k3 = p_3 + L_k3*(y3 - H_y3'*p_3);
p_k4 = p_4 + L_k4*(y4 - H_y4'*p_4);
p_k5 = p_5 + L_k5*(y5 - H_y5'*p_5);
p_k6 = p_6 + L_k6*(y6 - H_y6'*p_6);

%% Update covariance matrix
P_k1 = (eye(5) - L_k1*H_y1')*P1;
P_k2 = (eye(4) - L_k2*H_y2')*P2;
P_k3 = (eye(4) - L_k3*H_y3')*P3;
P_k4 = (eye(6) - L_k4*H_y4')*P4;
P_k5 = (eye(6) - L_k5*H_y5')*P5;
P_k6 = (eye(6) - L_k6*H_y6')*P6;

%% Re-initialize parameters for next time step
p_est1 = p_k1  ;    P1 = P_k1;
p_est2 = p_k2;      P2 = P_k2;
p_est3 = p_k3;      P3 = P_k3;
p_est4 = p_k4;      P4 = P_k4;
p_est5 = p_k5;      P5 = P_k5;
p_est6 = p_k6;      P6 = P_k6;

%% Output Model
y_est1 = H_y1'*p_k1;
y_est2 = H_y2'*p_k2;
y_est3 = H_y3'*p_k3;
y_est4 = H_y4'*p_k4;
y_est5 = H_y5'*p_k5;
y_est6 = H_y6'*p_k6;

%% Update Parameters
y       = [Cx;Cz;Cm;Cy;Cl;Cn];
y_est   = [y_est1;y_est2;y_est3;y_est4;y_est5;y_est6];
p_est   = [p_est1;p_est2;p_est3;p_est4;p_est5;p_est6];

%% Define Window Size
window = 100;
Innovation = y - y_est;

%% Define Aerodynamic Matrix
C_innovation_new = C_innovation(:,2:end);
C_innovation_new = horzcat(C_innovation_new, Innovation);

%% Calculate the Average of Innovation
avg = (1/window) * sum(C_innovation_new,2);

%% Calculate the Variance
var1 = 1/(window-1) * sum((C_innovation_new(1,:) - avg(1,:)).^2);
var2 = 1/(window-1) * sum((C_innovation_new(2,:) - avg(2,:)).^2);
var3 = 1/(window-1) * sum((C_innovation_new(3,:) - avg(3,:)).^2);
var4 = 1/(window-1) * sum((C_innovation_new(4,:) - avg(4,:)).^2);
var5 = 1/(window-1) * sum((C_innovation_new(5,:) - avg(5,:)).^2);
var6 = 1/(window-1) * sum((C_innovation_new(6,:) - avg(6,:)).^2);

%% Check for Failure
count_failure = 0;

if (var1/var_old(1)) > 10
    count_failure = count_failure + 1;
end
if (var2/var_old(2)) > 10
    count_failure = count_failure + 1;
end
if (var3/var_old(3)) > 10
    count_failure = count_failure + 1;
end
if (var4/var_old(4)) > 10
    count_failure = count_failure + 1;
end
if (var5/var_old(5)) > 10
    count_failure = count_failure + 1;
end
if (var6/var_old(6)) > 10
    count_failure = count_failure + 1;
end

if count_failure > 3
    trigger = 1;
else
    trigger = 0;
end
    
var_val = [var1;var2;var3;var4;var5;var6];
var_old = [var1;var2;var3;var4;var5;var6];

== matlab function Aerodynamic Model Identification/Variance ==
  data: Innovation input double; var_old input double; var output double; var_old output double; C_innovation input double; C_innovation output double; trigger input double; trigger output double
function [var,var_old,C_innovation, trigger] = variance(Innovation,var_old,C_innovation, trigger)
%% Define Window Size
window = 100;

%% Define Aerodynamic Matrix
C_innovation_new = C_innovation(:,2:end);
C_innovation_new = horzcat(C_innovation_new, Innovation);

%% Calculate the Average of Innovation
avg = (1/window) * sum(C_innovation_new,2);

%% Calculate the Variance
var1 = 1/(window-1) * sum((C_innovation_new(1,:) - avg(1,:)).^2);
var2 = 1/(window-1) * sum((C_innovation_new(2,:) - avg(2,:)).^2);
var3 = 1/(window-1) * sum((C_innovation_new(3,:) - avg(3,:)).^2);
var4 = 1/(window-1) * sum((C_innovation_new(4,:) - avg(4,:)).^2);
var5 = 1/(window-1) * sum((C_innovation_new(5,:) - avg(5,:)).^2);
var6 = 1/(window-1) * sum((C_innovation_new(6,:) - avg(6,:)).^2);

%% Check for Failure
count_failure = 0;
% var_old(1)
% var4
if (var4/var_old(1)) > 1.5
    count_failure = count_failure + 1;
end

if (var5/var_old(2)) > 1.5
    count_failure = count_failure + 1;
end

if (var6/var_old(3)) > 1.5
    count_failure = count_failure + 1;
end

if count_failure == 3
    trigger = 1;
else
    trigger = 0;
end
    
var = [var1;var2;var3;var4;var5;var6];
var_old = [var4;var5;var6];

%% Update Innovation Matrix
C_innovation = C_innovation_new;

== matlab function Aerodynamic Model Identification/Moving average square innovation ==
  data: Inputs input double; avg output double; C_list2 input double; C_list2 output double
function [avg,C_list2]= moving_avg(Inputs,C_list2)

%% Define Window Size
window = 100;

%% Define Aerodynamic Matrix
C_list_new = C_list2(:,2:end);
C_list_new = horzcat(C_list_new, Inputs);

%% Calculate Moving Average of Square Innovation
avg = 1/(window) * sum(C_list_new.^2,2);

%% Update new matrix
C_list2 = C_list_new;

== matlab function ANDI Rate Controller/b matrix ==
  data: inputs input double; states input double; rho input double; y output double; para input double
function y = b_matrix_andi(inputs,states,rho,para)
%% Define Parameters
Ixx = 11187.8;   b = 13.3250;   Vtas = states(4);
Iyy = 22854.8;   S = 24.9900;    
Izz = 31974.8;   c = 1.9910;     
Ixz = 1930.1;    m = 4500;       

%% Define RLS Parameters
CX0   = para(1);   CZ0  = para(6);    Cm0  = para(10); 
CXa   = para(2);   CZa  = para(7);    Cma  = para(11);
CXaa  = para(3);   CZq  = para(8);    Cmq  = para(12);
CXq   = para(4);   CZde = para(9);    Cmde = para(13);
CXde  = para(5);

CY0   = para(14);  Cl0   = para(20);  Cn0   = para(26);
CYb   = para(15);  Clb   = para(21);  Cnb   = para(27);
CYp   = para(16);  Clp   = para(22);  Cnp   = para(28);
CYr   = para(17);  Clr   = para(23);  Cnr   = para(29);
CYda  = para(18);  Clda  = para(24);  Cnda  = para(30);
CYdr  = para(19);  Cldr  = para(25);  Cndr  = para(31);

%% Define Matrices
I = [Ixx 0 -Ixz;
    0 Iyy 0;
    -Ixz 0 Izz];

M1 = [b*Clda 0 b*Cldr;
     0 c*Cmde 0;
     b*Cnda 0 b*Cndr];
 
%% Calculate B Matrix
B = (I./(0.5*rho*Vtas*Vtas*S)) * pinv(M1);
deflection = B*inputs;

y = deflection;

== matlab function ANDI Rate Controller/a matrix ==
  data: states input double; rho input double; y output double; para input double
function y = a_matrix(states,rho,para)
%% Define Parameters
Ixx = 11187.8;   b = 13.3250;   p    = states(1);   alpha = states(5);
Iyy = 22854.8;   S = 24.9900;   q    = states(2);   beta  = states(6);
Izz = 31974.8;   c = 1.9910;    r    = states(3);    
Ixz = 1930.1;    m = 4500;      Vtas = states(4); 

%% Define RLS Parameters
CX0   = para(1);   CZ0  = para(6);    Cm0  = para(10); 
CXa   = para(2);   CZa  = para(7);    Cma  = para(11);
CXaa  = para(3);   CZq  = para(8);    Cmq  = para(12);
CXq   = para(4);   CZde = para(9);    Cmde = para(13);
CXde  = para(5);

CY0   = para(14);  Cl0   = para(20);  Cn0   = para(26);
CYb   = para(15);  Clb   = para(21);  Cnb   = para(27);
CYp   = para(16);  Clp   = para(22);  Cnp   = para(28);
CYr   = para(17);  Clr   = para(23);  Cnr   = para(29);
CYda  = para(18);  Clda  = para(24);  Cnda  = para(30);
CYdr  = para(19);  Cldr  = para(25);  Cndr  = para(31);

%% Define Matrices
I = [Ixx 0 -Ixz;
    0 Iyy 0;
    -Ixz 0 Izz];

Cla = Cl0 + Clb*beta + Clp*(p*b/2*Vtas) + Clr*(r*b/2*Vtas);
Cma = Cm0 + Cma*alpha + Cmq*(q*c/Vtas);
Cna = Cn0 + Cnb*beta + Cnp*(p*b/2*Vtas) + Cnr*(r*b/2*Vtas);

M_rate = [p;q;r];
M_c    = [b*Cla;c*Cma;b*Cna];

%% Calculate A Matrix
A = -pinv(I) * (cross(M_rate, I*M_rate) + ((0.5*rho*Vtas^2*S) * M_c));
 
y = A;

== matlab function INDI Rate Controller/b matrix ==
  data: inputs input double; states input double; rho input double; y output double; para input double
function y = b_matrix_indi(inputs,states,rho,para)
%% Define Parameters
Ixx = 11187.8;   b = 13.3250;   Vtas = states(4);
Iyy = 22854.8;   S = 24.9900;    
Izz = 31974.8;   c = 1.9910;     
Ixz = 1930.1;    m = 4500;       

%% Define RLS Parameters
Clda = -0.1929; 
Cldr = -0.0000406;
Cmde = -0.9103;
Cnda = 0.05044;
Cndr = -0.06209;

%% Define Matrices
I = [Ixx 0 -Ixz;
    0 Iyy 0;
    -Ixz 0 Izz];

M1 = [b*Clda 0 b*Cldr;
     0 c*Cmde 0;
     b*Cnda 0 b*Cndr];
 
%% Calculate B Matrix
B = (I./(0.5*rho*Vtas*Vtas*S)) * pinv(M1);
deflection = B*inputs;

y = deflection;
